simulink model "mRobotArm_PickAndPlace"  (R2021a)
settings: Solver=FixedStepAuto  StartTime=0.0  StopTime=inf  RelTol=1e-3  EnableMultiTasking=on
undefined symbols (not defined in the file): adHome6deg, adHome6rad, adLinkLenghts, adMotorLimits, adWS, initPoint, pickPoint, pickPoint2, placePoint
libraries: arduinolib x17, aerolibconvert2 x3
settings Model: SILPILModeSetting=veronly  ExtModeTrigDuration=2  Creator=loris  LastModifiedBy=angelo
settings OptimizationCC: EnhancedBackFolding=on  PassReuseOutputArgsAs=Individual arguments  ZeroExternalMemoryAtStartup=off  ZeroInternalMemoryAtStartup=off  MaxStackSize=64  OptimizeBlockOrder=speed  DifferentSizesBufferReuse=on  OptimizationCustomize=off  EfficientTunableParamExpr=on
settings DebuggingCC: ParameterTunabilityLossMsg=error
settings HardwareCC: ProdBitPerInt=16  ProdBitPerPointer=16  ProdBitPerSizeT=16  ProdBitPerPtrDiffT=16  ProdLargestAtomicFloat=None  ProdWordSize=8  ProdHWDeviceType=Atmel->AVR
settings SFSimCC: MATLABDynamicMemAlloc=off
settings RTWCC: SystemTargetFile=ert.tlc  HardwareBoard=Arduino Mega 2560  TemplateMakefile=ert_default_tmf  Toolchain=Arduino AVR  BuildConfiguration=Faster Runs
settings CodeAppCC: ForceParamTrailComments=on  IgnoreCustomStorageClasses=off  OperatorAnnotations=on  SimulinkDataObjDesc=on  SFDataObjDesc=on  InsertBlockDesc=on
settings ERTTargetCC: SupportContinuousTime=on  SupportVariableSizeSignals=on  ExtModeStaticAllocSize=2048

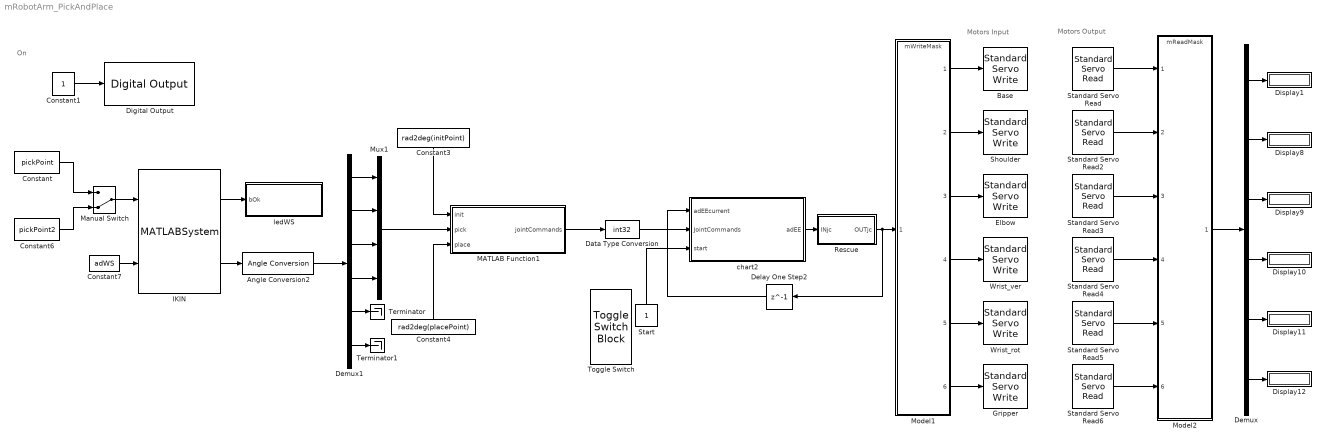
== system mRobotArm_PickAndPlace ==
  note: On
  note: Motors Output
  note: Motors Input
  Angle Conversion2 : aerolibconvert2/Angle Conversion  IU=rad  OU=deg
  Base : arduinolib/Standard Servo Write  pinNumber=11  ServoIndex=0  blockPlatform=ARDUINO
  Constant : Constant  Value=pickPoint
  Constant1 : Constant
  Constant3 : Constant  Value=rad2deg(initPoint)
  Constant4 : Constant  Value=rad2deg(placePoint)
  Constant6 : Constant  Value=pickPoint2
  Constant7 : Constant  Value=adWS
  Data Type Conversion : DataTypeConversion  OutDataTypeStr=int32  RndMeth=Round
  Delay One Step2 : Delay  DelayLength=1  InitialCondition=adHome6deg
  Demux : Demux  Outputs=6
  Demux1 : Demux  Outputs=6
  Digital Output : arduinolib/Digital Output  pinNumber=12  Direction=output  blockPlatform=arduino
  Display{1,8..12} (6 alike) : Display
  Elbow : arduinolib/Standard Servo Write  pinNumber=9  ServoIndex=1  blockPlatform=ARDUINO
  Gripper : arduinolib/Standard Servo Write  pinNumber=3  ServoIndex=2  blockPlatform=ARDUINO
  IKIN : MATLABSystem  System=oIKINSolver  adHomeDeg=adHome6deg  nGroundLength=adLinkLenghts(1)  nArmLength=adLinkLenghts(2)  nForearmLength=adLinkLenghts(3)  nHandLength=adLinkLenghts(4)  adBaseMinMaxDeg=adMotorLimits(1,:)  adShoulderMinMaxDeg=adMotorLimits(2,:)  adElbowMinMaxDeg=adMotorLimits(3,:)  adPitchMinMaxDeg=adMotorLimits(4,:)  adRollMinMaxDeg=adMotorLimits(5,:)  SimulateUsing=Code generation
      mask Type: oIKINSolver
      mask Display:
      | disp('oIKINSolver');
      | port_label('input',1,'adPoint');
      | port_label('input',2,'adWS');
      | port_label('output',1,'bFlag');
      | port_label('output',2,'adJC');
  MATLAB Function1 : MATLAB Function  TreatAsAtomicUnit=on
  Manual Switch : ManualSwitch  CurrentSetting=0
  Model1 : ModelReference  ModelNameDialog=mWriteMask.slx  SimulationMode=Normal  ModelReferenceVersion=1.6
  Model2 : ModelReference  ModelNameDialog=mReadMask.slx  SimulationMode=Normal  ModelReferenceVersion=1.7
  Mux1 : Mux
  Rescue : Subsystem
  Shoulder : arduinolib/Standard Servo Write  pinNumber=10  ServoIndex=3  blockPlatform=ARDUINO
  Standard Servo Read : arduinolib/Standard Servo Read  pinNumber=11  SampleTime=0.02  ServoIndex=0  blockPlatform=ARDUINO
      settings: SourceProductBaseCode=ARDUINO
  Standard Servo Read2 : arduinolib/Standard Servo Read  pinNumber=10  SampleTime=0.02  ServoIndex=3  blockPlatform=ARDUINO
      settings: SourceProductBaseCode=ARDUINO
  Standard Servo Read3 : arduinolib/Standard Servo Read  pinNumber=9  SampleTime=0.02  ServoIndex=1  blockPlatform=ARDUINO
      settings: SourceProductBaseCode=ARDUINO
  Standard Servo Read4 : arduinolib/Standard Servo Read  pinNumber=6  SampleTime=0.02  ServoIndex=4  blockPlatform=ARDUINO
      settings: SourceProductBaseCode=ARDUINO
  Standard Servo Read5 : arduinolib/Standard Servo Read  pinNumber=5  SampleTime=0.02  ServoIndex=5  blockPlatform=ARDUINO
      settings: SourceProductBaseCode=ARDUINO
  Standard Servo Read6 : arduinolib/Standard Servo Read  pinNumber=3  SampleTime=0.02  ServoIndex=2  blockPlatform=ARDUINO
      settings: SourceProductBaseCode=ARDUINO
  Start : Constant
  Terminator : Terminator
  Terminator1 : Terminator
  Toggle Switch : ToggleSwitchBlock  LabelPosition=Hide
      settings: Values={{'Off', 'On'}, [0 1]}
  Wrist_rot : arduinolib/Standard Servo Write  pinNumber=5  ServoIndex=5  blockPlatform=ARDUINO
  Wrist_ver : arduinolib/Standard Servo Write  pinNumber=6  ServoIndex=4  blockPlatform=ARDUINO
  chart2 : Stateflow chart  TreatAsAtomicUnit=on  SystemSampleTime=0.02
  ledWS : Subsystem  TreatAsAtomicUnit=on
  wires:
  Constant1/1 -> Digital Output/1
  Delay One Step2/1 -> chart2/1(adEEcurrent)
  Constant3/1 -> MATLAB Function1/1(init)
  Constant4/1 -> MATLAB Function1/3(place)
  Demux1/1 -> Mux1/1
  Demux1/2 -> Mux1/2
  Demux1/3 -> Mux1/3
  Demux1/4 -> Mux1/4
  Mux1/1 -> MATLAB Function1/2(pick)
  Demux1/5 -> Terminator/1
  chart2/1(adEE) -> Rescue/1(INjc)
  Start/1 -> chart2/3(start)
  Demux/6 -> Display12/1
  Demux/2 -> Display8/1
  Demux/5 -> Display11/1
  Demux/4 -> Display10/1
  Demux/1 -> Display1/1
  Demux/3 -> Display9/1
  Model2/1 -> Demux/1
  Demux1/6 -> Terminator1/1
  MATLAB Function1/1(jointCommands) -> Data Type Conversion/1
  Data Type Conversion/1 -> chart2/2(JointCommands)
  Model1/1 -> Base/1
  Model1/2 -> Shoulder/1
  Model1/3 -> Elbow/1
  Model1/4 -> Wrist_ver/1
  Model1/5 -> Wrist_rot/1
  Model1/6 -> Gripper/1
  Standard Servo Read/1 -> Model2/1
  Standard Servo Read2/1 -> Model2/2
  Standard Servo Read3/1 -> Model2/3
  Standard Servo Read4/1 -> Model2/4
  Standard Servo Read5/1 -> Model2/5
  Standard Servo Read6/1 -> Model2/6
  Rescue/1(OUTjc) -> Delay One Step2/1, Model1/1
  Constant/1 -> Manual Switch/1
  Constant6/1 -> Manual Switch/2
  Manual Switch/1 -> IKIN/1
  IKIN/1 -> ledWS/1(bOk)
  IKIN/2 -> Angle Conversion2/1
  Constant7/1 -> IKIN/2
  Angle Conversion2/1 -> Demux1/1

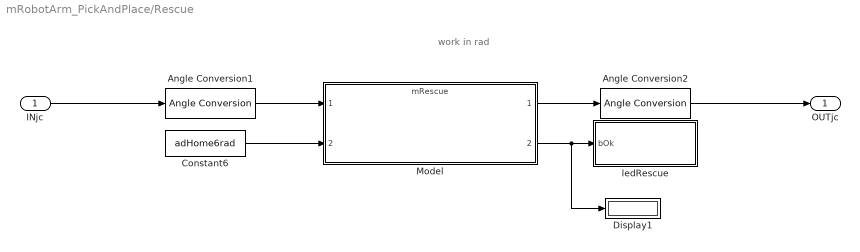
== system mRobotArm_PickAndPlace/Rescue ==
  note: work in rad
  INjc : Inport
  Angle Conversion1 : aerolibconvert2/Angle Conversion  IU=deg  OU=rad
  Angle Conversion2 : aerolibconvert2/Angle Conversion  IU=rad  OU=deg
  Constant6 : Constant  Value=adHome6rad
  Display1 : Display
  Model : ModelReference  ModelNameDialog=mRescue.slx  SimulationMode=Normal  ModelReferenceVersion=1.31
  ledRescue : Subsystem  TreatAsAtomicUnit=on
  OUTjc : Outport
  wires:
  Constant6/1 -> Model/2
  Angle Conversion1/1 -> Model/1
  INjc/1 -> Angle Conversion1/1
  Model/1 -> Angle Conversion2/1
  Angle Conversion2/1 -> OUTjc/1
  Model/2 -> Display1/1, ledRescue/1(bOk)

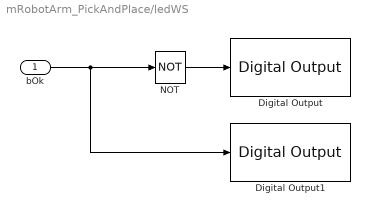
== system mRobotArm_PickAndPlace/ledWS ==
  bOk : Inport
  Digital Output : arduinolib/Digital Output  pinNumber=7  Direction=output  blockPlatform=arduino
  Digital Output1 : arduinolib/Digital Output  pinNumber=8  Direction=output  blockPlatform=arduino
  NOT : Logic  Operator=NOT  IconShape=distinctive  AllPortsSameDT=off  OutDataTypeStr=boolean
  wires:
  NOT/1 -> Digital Output/1
  bOk/1 -> Digital Output1/1, NOT/1

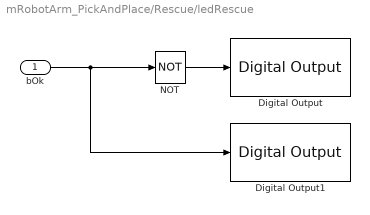
== system mRobotArm_PickAndPlace/Rescue/ledRescue ==
  bOk : Inport
  Digital Output : arduinolib/Digital Output  pinNumber=2  Direction=output  blockPlatform=arduino
  Digital Output1 : arduinolib/Digital Output  pinNumber=4  Direction=output  blockPlatform=arduino
  NOT : Logic  Operator=NOT  IconShape=distinctive  AllPortsSameDT=off  OutDataTypeStr=boolean
  wires:
  bOk/1 -> NOT/1, Digital Output1/1
  NOT/1 -> Digital Output/1

== stateflow chart mRobotArm_PickAndPlace/chart2 ==
  settings: executeAtInitialization=1
  state WayPoint1Reached
    entry:
    counter = 0;
    GripperDesired=50;
    during:
    adEE(6) = nextStep(adEEcurrent(6),GripperDesired);
    counter = temporalCount(sec);
  state Init
    entry:
    counter = 0;
    grip = 0;
    currentState=1;
    stop=0;
    GripperDesired=10;
    en:adEE = adEEcurrent;
    du:counter=temporalCount(sec);
  state ToNextState
    entry:
    if currentState<5
    currentState=currentState+1;
    else
    stop=1;
    adEE = adEEcurrent;
    end
    grip = 0;
  state Set
    entry:
    stop=0;
    counter=0;
    currentState=1;
    adEE(5) = 90;
    during:
    counter=temporalCount(sec);
  state WayPoint2Reached
    entry:
    counter = 0;
    GripperDesired=10;
    during:
    adEE(6) = nextStep(adEEcurrent(6),GripperDesired);
    counter = temporalCount(sec);
  state ToNextPoint
    entry:
    adEEdesired=JointCommands(currentState,:)';
    during:
    adEE = [
    nextStep(adEEcurrent(1), adEEdesired(1));
    nextStep(adEEcurrent(2), adEEdesired(2));
    nextStep(adEEcurrent(3), adEEdesired(3));
    nextStep(adEEcurrent(4), adEEdesired(4));
    adEE(5);
    adEE(6)];
  state CheckState
    entry:
    if currentState==2
    grip=1;
    elseif currentState==4
    grip=2;
    end
  WayPoint1Reached -> ToNextState : [counter>=5]
  (default) -> Init
  WayPoint2Reached -> ToNextState : [counter>=5]
  CheckState -> WayPoint1Reached [order 3] : [grip==1]
  ToNextState -> Set [order 2] : [stop==1]
  CheckState -> ToNextState [order 2] : [grip==0]
  Init -> Set : [counter > 1]
  ToNextState -> ToNextPoint [order 1] : [stop==0]
  Set -> ToNextPoint : [(counter>2) && (start==1)]
  CheckState -> WayPoint2Reached [order 1] : [grip==2]
  ToNextPoint -> CheckState : [all(adEEcurrent(1:4) == adEEdesired) ]
  data: current function_input; desired function_input; v function_output; current function_input; desired function_input; v function_output; current function_input; desired function_input; v function_output; adEEcurrent input; adEE output; adEEdesired local; currentState local; JointCommands input; stop local; start input; GripperDesired local; counter local; grip local
  function v = nextStep(current, desired):
    | function v = nextStep(current, desired)
    | if (current < desired)
    |     current = current + 1;
    | end
    | 
    | if (current > desired)
    |     current = current - 1;
    | end
    | 
    | v = current;
    | end
  function v = nextStep(current, desired):
    | function v = nextStep(current, desired)
    | if (current < desired)
    |     current = current + 1;
    | end
    | 
    | if (current > desired)
    |     current = current - 1;
    | end
    | 
    | v = current;
    | end
  function v = nextStep(current, desired):
    | function v = nextStep(current, desired)
    | if (current < desired)
    |     current = current + 1;
    | end
    | 
    | if (current > desired)
    |     current = current - 1;
    | end
    | 
    | v = current;
    | end

== matlab function mRobotArm_PickAndPlace/MATLAB Function1 ==
  data: init input; pick input; jointCommands output; place input
function jointCommands = compose(init, pick, place)
    jointCommands = [init'; pick'; init'; place'; init'];
end
